simulink model "LatTest"  (R2024b)
settings: Solver=ode4  StartTime=0.0  StopTime=30  FixedStep=0.01  RelTol=1e-3
undefined symbols (not defined in the file): fb_gain, fi_flag_Simulink, init_dlef, init_u_base, K_lat, x_ref_lat
settings Model: Creator=nefelibata  LastModifiedBy=nefelibata
settings DataIOCC: SaveState=on

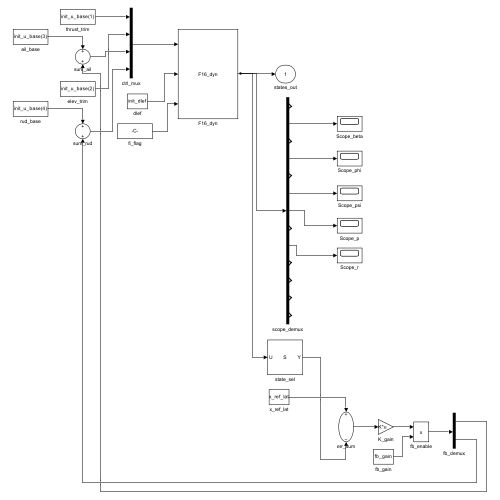
[thumbnail: Simulink's stored preview of the top-level diagram]
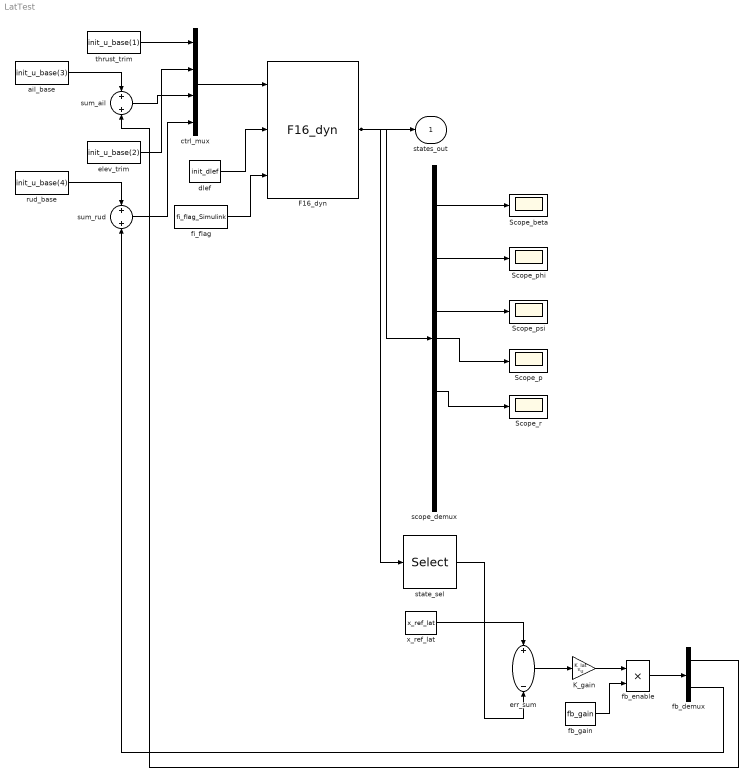
== system LatTest ==
  F16_dyn : S-Function  FunctionName=F16_dyn  Parameters=init_x  SFunctionDeploymentMode=off  EnableBusSupport=off
  K_gain : Gain  Gain=K_lat  Multiplication=Matrix(K*u)
  Scope_beta : Scope
  Scope_p : Scope
  Scope_phi : Scope
  Scope_psi : Scope
  Scope_r : Scope
  ail_base : Constant  Value=init_u_base(3)
  ctrl_mux : Mux
  dlef : Constant  Value=init_dlef
  elev_trim : Constant  Value=init_u_base(2)
  err_sum : Sum  Inputs=+-
  fb_demux : Demux  Outputs=2
  fb_enable : Product  Inputs=**
  fb_gain : Constant  Value=fb_gain
  fi_flag : Constant  Value=fi_flag_Simulink
  rud_base : Constant  Value=init_u_base(4)
  scope_demux : Demux  Outputs=13
  state_sel : Selector  InputPortWidth=13  IndexOptions=Index vector (dialog)  Indices=[2,4,6,7,9]  OutputSizes=1
  sum_ail : Sum
  sum_rud : Sum
  thrust_trim : Constant  Value=init_u_base(1)
  x_ref_lat : Constant  Value=x_ref_lat
  states_out : Outport
  wires:
  ail_base/1 -> sum_ail/1
  sum_rud/1 -> ctrl_mux/4
  rud_base/1 -> sum_rud/1
  sum_ail/1 -> ctrl_mux/3
  elev_trim/1 -> ctrl_mux/2
  thrust_trim/1 -> ctrl_mux/1
  x_ref_lat/1 -> err_sum/1
  dlef/1 -> F16_dyn/2
  fb_gain/1 -> fb_enable/2
  fi_flag/1 -> F16_dyn/3
  ctrl_mux/1 -> F16_dyn/1
  F16_dyn/1 -> state_sel/1, states_out/1, scope_demux/1
  scope_demux/6 -> Scope_psi/1
  scope_demux/2 -> Scope_beta/1
  scope_demux/4 -> Scope_phi/1
  scope_demux/7 -> Scope_p/1
  scope_demux/9 -> Scope_r/1
  err_sum/1 -> K_gain/1
  state_sel/1 -> err_sum/2
  K_gain/1 -> fb_enable/1
  fb_demux/2 -> sum_rud/2
  fb_enable/1 -> fb_demux/1
  fb_demux/1 -> sum_ail/2
